simulink model "L3_T1_dq_pmsm"  (R2026a)
settings: Solver=ode23tb  StartTime=0  StopTime=40  MaxStep=0.002
settings Model: Creator=m  LastModifiedBy=m

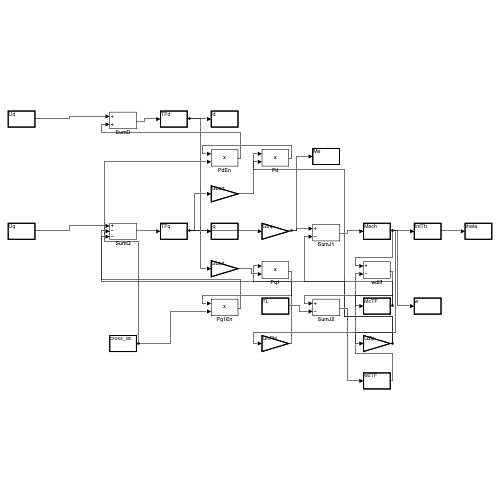
[thumbnail: Simulink's stored preview of the top-level diagram]
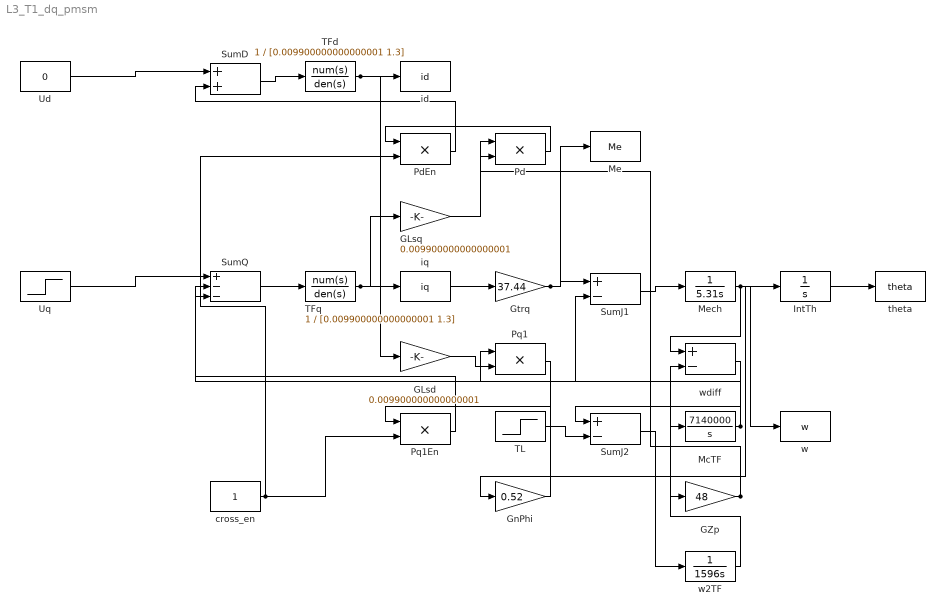
== system L3_T1_dq_pmsm ==
  GLsd : Gain  Gain=0.009900000000000001
  GLsq : Gain  Gain=0.009900000000000001
  GZp : Gain  Gain=48
  GnPhi : Gain  Gain=0.52
  Gtrq : Gain  Gain=37.44
  IntTh : Integrator
  McTF : TransferFcn  Numerator=7140000  Denominator=[1 0]
  Me : ToWorkspace  VariableName=Me  SaveFormat=Structure With Time  SampleTime=-1
  Mech : TransferFcn  Numerator=1  Denominator=[5.31 0]
  Pd : Product
  PdEn : Product
  Pq1 : Product
  Pq1En : Product
  SumD : Sum
  SumJ1 : Sum  Inputs=+-
  SumJ2 : Sum  Inputs=+-
  SumQ : Sum  Inputs=+--
  TFd : TransferFcn  Numerator=1  Denominator=[0.009900000000000001 1.3]
  TFq : TransferFcn  Numerator=1  Denominator=[0.009900000000000001 1.3]
  TL : Step  Time=20  FinalValue=100  SampleTime=0
  Ud : Constant  Value=0
  Uq : Step  Time=0  FinalValue=380.9113043478261  SampleTime=0
  cross_en : Constant
  id : ToWorkspace  VariableName=id  SaveFormat=Structure With Time  SampleTime=-1
  iq : ToWorkspace  VariableName=iq  SaveFormat=Structure With Time  SampleTime=-1
  theta : ToWorkspace  VariableName=theta  SaveFormat=Structure With Time  SampleTime=-1
  w : ToWorkspace  VariableName=w  SaveFormat=Structure With Time  SampleTime=-1
  w2TF : TransferFcn  Numerator=1  Denominator=[1596 0]
  wdiff : Sum  Inputs=+-
  wires:
  SumD/1 -> TFd/1
  SumQ/1 -> TFq/1
  TFq/1 -> Gtrq/1, GLsq/1, iq/1
  Gtrq/1 -> SumJ1/1, Me/1
  SumJ1/1 -> Mech/1
  Mech/1 -> wdiff/1, GZp/1, IntTh/1, w/1
  w2TF/1 -> wdiff/2
  wdiff/1 -> McTF/1
  McTF/1 -> SumJ1/2, SumJ2/1
  SumJ2/1 -> w2TF/1
  GZp/1 -> Pd/1, Pq1/1, GnPhi/1
  GLsq/1 -> Pd/2
  Pd/1 -> PdEn/1
  cross_en/1 -> PdEn/2, Pq1En/2
  PdEn/1 -> SumD/2
  TFd/1 -> GLsd/1, id/1
  GLsd/1 -> Pq1/2
  Pq1/1 -> Pq1En/1
  Pq1En/1 -> SumQ/2
  GnPhi/1 -> SumQ/3
  Ud/1 -> SumD/1
  Uq/1 -> SumQ/1
  TL/1 -> SumJ2/2
  IntTh/1 -> theta/1
